simulink model "ThreeDOF_SMA_Spring_Hand"  (R2021b)
settings: Solver=FixedStepAuto  StartTime=0.0  StopTime=1.5  FixedStep=.001  RelTol=1e-3
libraries: RCTblocks x1
settings Model: Creator=Spino.shop  LastModifiedBy=Spino.shop
settings SFSimCC: SimTargetLang=C++

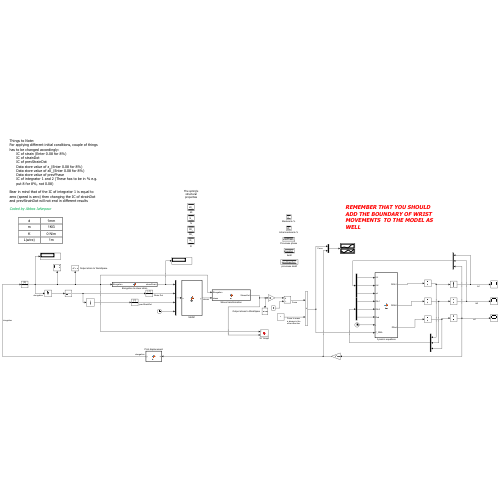
[thumbnail: Simulink's stored preview of the top-level diagram]
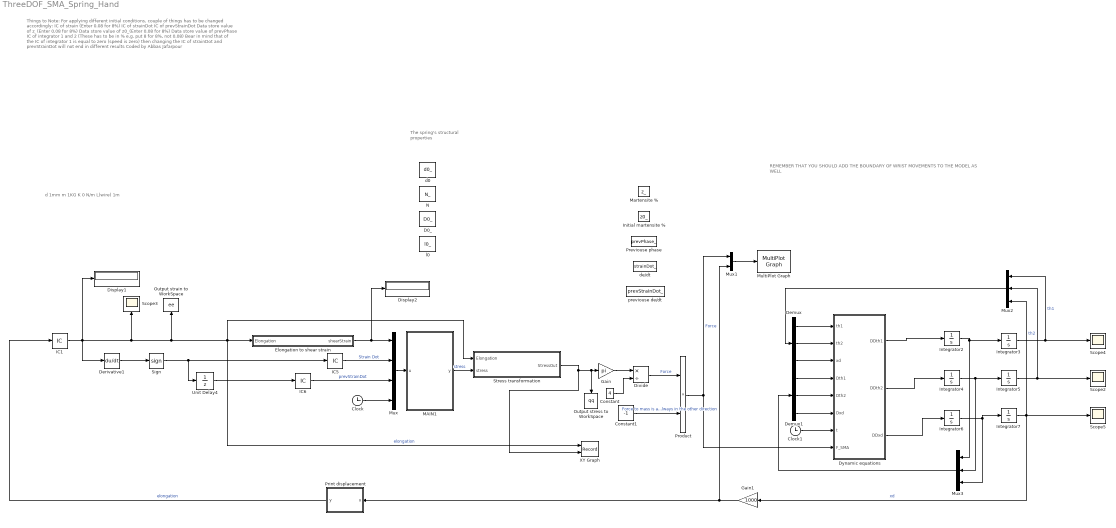
== system ThreeDOF_SMA_Spring_Hand ==
  note: Things to Note:
      | For applying different initial conditions, couple of things has to be changed accordingly:
      | IC of strain (Enter 0.08 for 8%)
      | IC of strainDot
      | IC of prevStrainDot
      | Data store value of z_(Enter 0.08 for 8%)
      | Data store value of z0_(Enter 0.08 for 8%)
      | Data store value of prevPhase
      | IC of integrator 1 and 2 (These has to be in % e.g. put 8 for 8%, not 0.08)
      |
      | Bear in mind that of the IC of integrator 1 is equal to zero (speed is zero) then changing the IC of strainDot and prevStrainDot will not end in different results
      |
      | Coded by Abbas Jafarpour
  note: d
      | 1mm
      |
      | m
      | 1KG
      |
      | K
      | 0 N/m
      |
      | L(wire)
      | 1m
  note: The spring's structural properties
  note: REMEMBER THAT YOU SHOULD ADD THE BOUNDARY OF WRIST MOVEMENTS TO THE MODEL AS WELL
  Clock : Clock
  Clock1 : Clock
  Constant : Constant  Value=4
  Constant1 : Constant  Value=-1
  D0_ : DataStoreMemory  DataStoreName=D0_  ReadBeforeWriteMsg=warning  WriteAfterWriteMsg=warning  WriteAfterReadMsg=warning  InitialValue=7.3  VectorParams1D=off  ShowAdditionalParam=off  OutDataTypeStr=double
  Demux : Demux  Outputs=3
  Demux1 : Demux  Outputs=3
  Derivative1 : Derivative
  Display1 : Display
  Display2 : Display
  Divide : Product  Inputs=*/
  Dynamic equations : MATLAB Function  TreatAsAtomicUnit=on
  Elongation to shear strain : MATLAB Function  TreatAsAtomicUnit=on
  Gain : Gain  Gain=pi
  Gain1 : Gain  Gain=1000
  IC1 : InitialCondition  Value=0
  IC5 : InitialCondition  Value=-1
  IC6 : InitialCondition  Value=-1
  Initial martensite % : DataStoreMemory  DataStoreName=z0_  ReadBeforeWriteMsg=warning  WriteAfterWriteMsg=warning  WriteAfterReadMsg=warning  InitialValue=1  ShowAdditionalParam=off  OutDataTypeStr=double
  Integrator{2..7} (6 alike) : Integrator
  MAIN1 : MATLAB Function  TreatAsAtomicUnit=on
  Martensite % : DataStoreMemory  DataStoreName=z_  ReadBeforeWriteMsg=warning  WriteAfterWriteMsg=warning  WriteAfterReadMsg=warning  InitialValue=0.015  ShowAdditionalParam=off  OutDataTypeStr=double
  MultiPlot Graph : RCTblocks/MultiPlot Graph  Tag=MultiPlot  tmin=0  tmax=1.5  ymin=-40  ymax=40  Tsamp=-1  vnamesave=multisimout
      settings: SourceProductBaseCode=RC
  Mux : Mux
  Mux1 : Mux  Inputs=2
  Mux2 : Mux  Inputs=3
  Mux3 : Mux  Inputs=3
  N : DataStoreMemory  DataStoreName=N_  ReadBeforeWriteMsg=warning  WriteAfterWriteMsg=warning  WriteAfterReadMsg=warning  InitialValue=5  ShowAdditionalParam=off  OutDataTypeStr=double
  Output strain to WorkSpace : ToWorkspace  VariableName=ee  SampleTime=-1
      settings: Save2DSignal=2-D array (concatenate along first dimension)
  Output stress to WorkSpace : ToWorkspace  VariableName=qq  SampleTime=-1
      settings: Save2DSignal=2-D array (concatenate along first dimension)
  Previouse phase : DataStoreMemory  DataStoreName=prevPhase_  ReadBeforeWriteMsg=warning  WriteAfterWriteMsg=warning  WriteAfterReadMsg=warning  InitialValue=5  ShowAdditionalParam=off  OutDataTypeStr=double
  Print displacement : MATLAB Function  TreatAsAtomicUnit=on
  Product : Product
  Scope{2..5} (4 alike) : Scope
  Sign : Signum
  Stress transformation : MATLAB Function  TreatAsAtomicUnit=on
  Unit Delay4 : UnitDelay  SampleTime=-1  HasFrameUpgradeWarning=on
  XY Graph : Record  FileSettingsInternal="{\"entries\":[{\"content\":{\"excelSettings\":{\"content\":{},\"type\":\"Streamout.ExcelSettings\"}},\"type\":\"Streamout.FileSettingStorage\",\"uuid\":\"8585d984-787d-4496-8735-ede648e09058\"}],\"packageUris\":[\"http://schema.mathworks.com/mf0/streamout_blocks/R2020a\"],\"version\":\"1.0\"}"  Layout=[1 1]  SignalsInternal="{\"entries\":[{\"content\":{\"signals\":[{\"content\":{\"blockPath\":[\"ThreeDOF_SMA_Spring_Hand/XY Graph\"],\"channel\":[],\"dimensions\":[1],\"domain\":\"ThreeDOF_SMA_Spring_Hand/XY Graph\",\"lineColor\":\"#a2142f\",\"plots\":[1],\"port\":1,\"sid\":[],\"signalID\":9,\"signalName\":\"elongation\"},\"type\":\"RecordBlkView.Signal\",\"uuid\":\"1176787e-02b1-4e58-a8f1-352873b659ce\"},{\"content\":{\"blockPath\":[\"ThreeDOF_SMA_Spring_Hand/XY Graph\"],\"channel\":[],\"dimensions\":[1],\"domain\":\"ThreeDOF_SMA_Spring_Hand/XY Graph\",\"lineColor\":\"#139fff\",\"plots\":[1],\"port\":2,\"sid\":[],\"signalID\":12,\"signalName\":\"Stress transformation\"},\"type\":\"RecordBlkView.Signal\",\"uuid\":\"6b0ce42b-1ab9-4c2f-8a20-9cf08699349f\"}]},\"type\":\"RecordBlkView.InputSignals\",\"uuid\":\"cd44c269-2911-4699-ac86-e4ccbff490f5\"}],\"packageUris\":[\"http://schema.mathworks.com/mf0/streamout_blocks/R2020a\"],\"version\":\"1.0\"}"  VisualizationBindings="{\"xyplotplugin\":{\"info\":[{\"series\":[{\"bindingParametersList\":[{\"parameter\":\"X-Axis\",\"signalID\":9,\"signalName\":\"elongation\"},{\"parameter\":\"Y-Axis\",\"signalID\":12,\"signalName\":\"Stress transformation\"}],\"seriesID\":6978}],\"subplotID\":1}]}}"  CompatibilityTag=XY
  d0 : DataStoreMemory  DataStoreName=d0_  ReadBeforeWriteMsg=warning  WriteAfterWriteMsg=warning  WriteAfterReadMsg=warning  InitialValue=1  ShowAdditionalParam=off  OutDataTypeStr=double
  de/dt : DataStoreMemory  DataStoreName=strainDot_  ReadBeforeWriteMsg=warning  WriteAfterWriteMsg=warning  WriteAfterReadMsg=warning  InitialValue=1  ShowAdditionalParam=off  OutDataTypeStr=double
  l0 : DataStoreMemory  DataStoreName=l0_  ReadBeforeWriteMsg=warning  WriteAfterWriteMsg=warning  WriteAfterReadMsg=warning  InitialValue=5  ShowAdditionalParam=off  OutDataTypeStr=double
  previouse de/dt : DataStoreMemory  DataStoreName=prevStrainDot_  ReadBeforeWriteMsg=warning  WriteAfterWriteMsg=warning  WriteAfterReadMsg=warning  InitialValue=1  ShowAdditionalParam=off  OutDataTypeStr=double
  wires:
  Unit Delay4/1 -> IC6/1
  Mux/1 -> MAIN1/1(u)
  Derivative1/1 -> Sign/1
  Clock/1 -> Mux/4
  Sign/1 -> Unit Delay4/1, IC5/1
  Gain/1 -> Divide/1
  Constant/1 -> Divide/2
  IC1/1 -> Scope3/1, Output strain to WorkSpace/1, Stress transformation/1(Elongation), XY Graph/1, Elongation to shear strain/1(Elongation), Derivative1/1, Display1/1  "elongation"
  IC5/1 -> Mux/2  "Strain Dot"
  IC6/1 -> Mux/3  "prevStrainDot"
  Divide/1 -> Product/1  "Force"
  Product/1 -> Dynamic equations/8(F_SMA), Mux1/1  "Force"
  Mux1/1 -> MultiPlot Graph/1
  Constant1/1 -> Product/2  "Force to mass is always in the other direction"
  Print displacement/1(y) -> IC1/1  "elongation"
  MAIN1/1(y) -> Stress transformation/2(stress)  "stress"
  Stress transformation/1(StressOut) -> XY Graph/2, Output stress to WorkSpace/1, Gain/1
  Elongation to shear strain/1(shearStrain) -> Display2/1, Mux/1
  Gain1/1 -> Mux1/2, Print displacement/1(u)
  Integrator2/1 -> Mux3/1, Integrator3/1
  Integrator6/1 -> Integrator7/1, Mux3/3
  Demux1/1 -> Dynamic equations/4(Dth1)
  Demux/3 -> Dynamic equations/3(xd)
  Mux2/1 -> Demux/1
  Demux1/2 -> Dynamic equations/5(Dth2)
  Integrator3/1 -> Scope4/1, Mux2/1  "th1"
  Dynamic equations/3(DDxd) -> Integrator6/1
  Demux/2 -> Dynamic equations/2(th2)
  Mux3/1 -> Demux1/1
  Demux/1 -> Dynamic equations/1(th1)
  Clock1/1 -> Dynamic equations/7(t)
  Integrator7/1 -> Gain1/1, Mux2/3, Scope5/1  "xd"
  Integrator5/1 -> Scope2/1, Mux2/2  "th2"
  Dynamic equations/1(DDth1) -> Integrator2/1
  Integrator4/1 -> Mux3/2, Integrator5/1
  Dynamic equations/2(DDth2) -> Integrator4/1
  Demux1/3 -> Dynamic equations/6(Dxd)

== matlab function ThreeDOF_SMA_Spring_Hand/Elongation to shear strain ==
  settings: updateMethod=DISCRETE
  data: shearStrain output; Elongation input; N_ data_store_memory; d0_ data_store_memory; D0_ data_store_memory; l0_ data_store_memory
% Because we have Nonlinear shera transformation in the entire
% crosssection, to avoide unncessary complexity we take shear as a linear
% function in the wire's crossection and approximate the integral. Refer to
% the paper for proof of the formula and the way we acquire these
% parameters.
function shearStrain = fcn(Elongation)
    
    % Processing the grlobal variables
    global D0_ d0_ l0_ N_;
    D0 = D0_;
    N = N_;
    d0 = d0_;
    l0 = l0_;

    R0 = D0/2;
    r0 = d0/2;

    alpha0 = atan(l0 / (2 * pi * N * R0) ); % Initial helix angle
    L = sqrt(l0 + (2 * pi * N * R0)^2); % The total length of the spring 
    
    r0  = d0 / 2;
    alpha = asin( Elongation / L + sin(alpha0) );
    R = R0 * cos(alpha) / cos(alpha0);
    
    shearStrain = Elongation * r0 / (2 * pi * N * R^2) * (3/4);
end

== matlab function ThreeDOF_SMA_Spring_Hand/Print displacement ==
  data: u input; y output
function y = fcn(u)
    y = u;
    fprintf("====>> displacement : %.5f\n",u);
end

== matlab function ThreeDOF_SMA_Spring_Hand/Stress transformation ==
  settings: updateMethod=DISCRETE
  data: Elongation input; stress input; StressOut output; N_ data_store_memory; l0_ data_store_memory; D0_ data_store_memory; d0_ data_store_memory
function StressOut = fcn(Elongation, stress)

    % Processing the grlobal variables
    global D0_ d0_ l0_ N_;
    D0 = D0_;
    N = N_;
    d0 = d0_;
    l0 = l0_;

    R0 = D0/2;
    r0 = d0/2;

    alpha0 = atan(l0 / (2 * pi * N * R0) ); % Initial helix angle
    L = sqrt(l0 + (2 * pi * N * R0)^2); % The total length of the spring 
    
    % Calculating the spring diameter change
    alpha = asin( Elongation / L + sin(alpha0) );
    R = R0 * cos(alpha) / cos(alpha0);

    StressOut = stress * 2 * pi * r0 ^ 3 / 3 / R;
end

== matlab function ThreeDOF_SMA_Spring_Hand/Dynamic equations ==
  data: th1 input; th2 input; xd input; Dth1 input; Dth2 input; Dxd input; DDth1 output; DDth2 output; DDxd output; t input; F_SMA input
function [DDth1, DDth2, DDxd] = fcn(th1, th2, xd, Dth1, Dth2, Dxd, t, F_SMA)

T1 = sin(t);
T2 = cos(t);


Y = zeros(6,1);
Y(1) = xd;
Y(2) = Dxd;
Y(3) = th1;
Y(4) = Dth1;
Y(5) = th2;
Y(6) = Dth2;

DDxd = -(3*F_SMA - T1 + cos(Y(3) - Y(5))^2*Y(2) - cos(Y(5))*cos(Y(3) - Y(5)) + sin(Y(3) - Y(5))*Y(6)^2 ...
    - sin(Y(3))*Y(1) + T2*cos(Y(3) - Y(5)) + cos(Y(3))*cos(Y(3) - Y(5))^2 - F_SMA*cos(Y(3) - Y(5))^2 ...
    - cos(Y(3) - Y(5))*Y(5) - cos(Y(3) - Y(5))*Y(6) - 3*Y(2) + Y(3) + Y(4) + ...
    cos(Y(3) - Y(5))*sin(Y(3) - Y(5))*Y(4)^2)/(cos(Y(3) - Y(5))^2 - 2);

DDth1 = (F_SMA - T1 + 2*cos(Y(3)) - cos(Y(5))*cos(Y(3) - Y(5)) + sin(Y(3) - Y(5))*Y(6)^2 - sin(Y(3))*Y(1) ...
    + T2*cos(Y(3) - Y(5)) - cos(Y(3) - Y(5))*Y(5) - cos(Y(3) - Y(5))*Y(6) - Y(2) + Y(3) + Y(4) + ...
    cos(Y(3) - Y(5))*sin(Y(3) - Y(5))*Y(4)^2)/(cos(Y(3) - Y(5))^2 - 2);

DDth2 = -(2*T2 - 2*cos(Y(5)) + 2*cos(Y(3))*cos(Y(3) - Y(5)) + 2*sin(Y(3) - Y(5))*Y(4)^2 + ...
    F_SMA*cos(Y(3) - Y(5)) - T1*cos(Y(3) - Y(5)) - cos(Y(3) - Y(5))*Y(2) + cos(Y(3) - Y(5))*Y(3) ...
    + cos(Y(3) - Y(5))*Y(4) - 2*Y(5) - 2*Y(6) + cos(Y(3) - Y(5))*sin(Y(3) - Y(5))*Y(6)^2 ...
    - sin(Y(3))*cos(Y(3) - Y(5))*Y(1))/(cos(Y(3) - Y(5))^2 - 2);

== matlab function ThreeDOF_SMA_Spring_Hand/MAIN1 ==
  settings: updateMethod=DISCRETE
  data: u input; y output; z_ data_store_memory; z0_ data_store_memory; prevPhase_ data_store_memory; d0_ data_store_memory; D0_ data_store_memory; l0_ data_store_memory; N_ data_store_memory
function y = fcn(u)

    % Processing the grlobal variables for Material structural
    % properties
    global D0_ d0_ l0_ N_;
    D0 = D0_; % Wire diameter (mm)
    N = N_  ; % Number of coils
    d0 = d0_; % Coil diameter (mm) 
    l0 = l0_; % Initial length of spring l0 (mm) 
        
    % Processing the grlobal variables for SMA phase and strain
    global z_ z0_ strainDot_ prevStrainDot_ prevPhase_;

    % Initiate material properties
    X = 6;
    if false
        kj = 1;
    elseif X == 6
        Mf = 9; Ms = 18.4; As = 34.5; Af = 49;
    
        CA_Loading = 13.8; CA_Unloading = 13.8;
        CM_Loading = 8   ; CM_Unloading = 8   ; 
        critStressFinish = 170; critStressStart = 100;
    
        Ga = 67e3; Gm = 26.3e3; eL = 0.067;
        T = 60;
    
        S_M_finish_Loading = critStressFinish + CM_Loading*(T-Ms); S_M_finish_Unloading = critStressFinish + CM_Unloading*(T-Ms);
        S_M_start_Loading = critStressStart + CM_Loading*(T-Ms); S_M_start_Unloading = critStressStart + CM_Unloading*(T-Ms);
        S_A_start_Loading = CA_Loading*(T-As); S_A_start_Unloading = CA_Unloading*(T-As);
        S_A_finish_Loading = CA_Loading*(T-Af); S_A_finish_Unloading = CA_Unloading*(T-Af);
    
        S_M_finish = [S_M_finish_Loading S_M_finish_Unloading];
        S_M_start = [S_M_start_Loading S_M_start_Unloading];
        S_A_start = [S_A_start_Loading S_A_start_Unloading];
        S_A_finish = [S_A_finish_Loading S_A_finish_Unloading];
    end


    y = 0;

    strain = u(1); eDot = u(2); prevStrainDot = u(3);
    
    % When eDot is zero, change eDot to previouse eDot
    if eDot == 0
        eDot = prevStrainDot;
    end

    % We get eDot from derivative of e with respect to time, on negative
    % strains this causes the code to think that we are unloading while
    % actually we are loading. we solve this by conditions below
    if(strain < 0 && eDot < 0)
        eDot = 1;
    elseif(strain < 0 && eDot > 0)
        eDot = -1;
    end

    % Do the same for previouse step's strainDot
    if(strain < 0 && prevStrainDot < 0)
        prevStrainDot = 1;
    elseif(strain < 0 && prevStrainDot > 0)
        prevStrainDot = -1;
    end

    fprintf("\n\nMAIN (%.4fs); z0:%.4f ||z:%.4f ||strain:%.5f || strainDot: %.1f || prevStrainDot: %.1f ||prevPhase:%.1f || \n",u(4), z0_,z_,strain,eDot,prevStrainDot,prevPhase_);
    % Note that: [z0,z,previousePahse,stress] --> [y(1),y(2),y(3),y(4)]

    [z0_,z_,prevPhase_,y] = MAIN(z0_,z_,prevPhase_,strain,eDot, prevStrainDot,T,eL,Gm,Ga,Ms,As, S_M_finish, S_M_start, S_A_finish, S_A_start);
    
    fprintf("One pass done.")

    y = double(y);

end

function [z0,z,phase,stress] = MAIN(z0,z,previousePahse,strain,strainDot, prevStrainDot,T,eL,Gm,Ga,Ms,As, S_M_finish, S_M_start, S_A_finish, S_A_start)
    coder.extrinsic("stressFinder");

    %This function with strain as an input and some other inputs, returns
    %stress and some other variables (These variables are used as inputs for the next iteration)
    %This function helps us avoide doing the calculations inside the loop
    %INPUTS:
    %z0: The martensite ratio at start of previouse phase
    %z: The martensite ratio of previouse iteration (It is different form z0)
    %prevPhase: The phase of previouse iteration
    %strain: Current strain
    %strainDot: Current strain rate

    %Only pseudoelastic
    zT = 0; zT0 = 0;

    %When we reverse in the middle of phase transformation, we need to
    %update z0, but due to us not having the stress, we cant know if we
    %have changed phase (phaseFinder function needs stress as an input)
    %to solve this error, we know if we have reversed if previose eDot
    %is not equal to current eDot. when they are not equal, we update
    %the value of z0
    reverse = false;
    if prevStrainDot ~= strainDot
        reverse = true;
    end

    if reverse
        zS0 = z;
        z0 = z;
    end
    
    % Passing different critical stress's to required functions for loading
    % and unlaoding. This helps us to adopt for the simulations that CM and
    % CA are different for loading and unloading
    if 0 <= strainDot
        i = 1;
    else
        i = 2;
    end

    stress = 0;
    stress = stressFinder(previousePahse, strain, strainDot, T, eL, Gm, Ga, z0, zT, S_M_finish(i), S_M_start(i), S_A_finish(i), S_A_start(i));

    phase = phaseFinder(previousePahse, stress, strainDot,z,z0, S_M_finish(i), S_M_start(i), S_A_finish(i), S_A_start(i));
    fprintf("Current phase: %.1f\n",phase);
    if previousePahse ~= phase
        phaseChange = true;
        fprintf("ER1\n");
    else
        phaseChange = false;
    end
    
    %When we finsh phase 2 and go to phase 3 z is not exactly equal to
    %1, this causes errors in stressFinder function, so by this line we
    %fix this
    if (previousePahse == 2 && phase == 3) || (previousePahse == 222 && phase == 3) 
        z = 1;
    elseif (previousePahse == 5 && phase == 6) 
        z = 0;
    end
    
    if phaseChange
        fprintf("ER2\n");
        zS0 = z;
        z0 = z;
    end

    %The get_z function cant process negative stresses, so we multiply the
    %stress by -1 and at the end we change it back
    if(strain < 0)
        fprintf("ER3\n");
        NEGATIVESTRAIN = true;
        stress = stress * -1;
    end

    z = get_z(stress,strainDot,T,Ms,As,z0,zT,z, S_M_finish(i), S_M_start(i), S_A_finish(i), S_A_start(i));
    
    %Change back
    if(strain < 0)
        fprintf("ER4\n");
        NEGATIVESTRAIN = true;
        stress = stress * -1;
    end

    z = double(z);
    z0 = double(z0);
    stress = double(stress);
end


function [phase] = phaseFinder(prevPhase, stress, strainDot,z,z0, S_M_finish, S_M_start, S_A_finish, S_A_start)
    %Note that due to nature of my project zT is always equal to zero and we can use z instead of zS
    stress = double(stress);

    %This function returns the SMA's phase number in pseudoelastic a
    %procedure with Brinsons's (1993 and 1996) constitutive modeling
    %Phase Numbering:
    %loading before phase change : 1  || loading with phase change : 2  || loading after phase change : 3 
    %unloading before phase change : 4  || unloading with phase change : 5  || unloading after phase change : 6 
    %Phases for handeling inner loops are:
    %Loading while in middle of Martensite->Austenite phase change: 8
    %Loading when below martensit transformation start stress while  z != 0: 9
    %Loading while coming back into austenite phase Chaneg area while  z !=0: 10
    %**Note that the phases that are caused from reversals in loading in the middle of  a phase are repeated numers (e.g. 77 or 11)
    %Unloading before Austenite has changed to martensite (reversing in middle of phase 1):11
    %Unloading while in middle of Austenite->Martensite phase change: 22
    %Reversing phase 7 and continuing loading:77
    %Reversing in middle of phase 5 and continuing loading:55
    %
    %
    %For defining the inner loops we also need to know where we came from,
    %so we need the previous step's direction (loading or unloading)
    %* Note that stressDot is the direction of loading, +1 for loading and
    %-1 for unloading

    %UPDATE: some times, we have negative strain. In order for this
    %function to handle that, we define This constant. if it is true, all
    %the calculations will be in positive numbers but at the end they will
    %be multiplied by -1
    NEGATIVESTRAIN = false;
    
    if(stress < 0)
        NEGATIVESTRAIN = true;
        stress = stress * -1;
    end

    phase = -1;
    if (S_M_start < stress && stress < S_M_finish) && 0 < strainDot && z0 == 0
        phase = 2;
    elseif not(S_M_start < stress && stress < S_M_finish) && (stress < S_M_start) && 0 < strainDot && z == 0
        phase = 1;
    elseif not(S_M_start < stress && stress < S_M_finish) && (S_M_finish < stress) && 0 < strainDot
        phase = 3;
    elseif not( S_A_finish < stress && stress < S_A_start  ) && strainDot < 0 && (S_A_start < stress)  && z == 1
        phase = 4;
    elseif ( S_A_finish < stress && stress < S_A_start  ) && strainDot < 0 && 0 < z
        phase = 5;
    elseif not( S_A_finish < stress && stress < S_A_start  ) && strainDot < 0  && (stress < S_A_finish) && prevPhase ~= 11
        %Some times we start unloading while in phase 1, so to
        %differenciate this with phase 6, we have to make a new phase and
        %"&& prevPhase ~= 1" condition as well. to avoid devision by zero
        %add
        phase = 6;
    elseif not(S_M_start < stress && stress < S_M_finish) && (stress < S_M_start) && strainDot < 0 && z == 0
        %Unloading before Austenite has changed to martensite (reversing in middle of phase 1)
        phase = 11;
    elseif (z0 < 1) && (stress < S_M_finish) && (S_A_start < stress) && strainDot < 0
        %Inner loop: Unloading while in middle of Austenite->Martensite phase change
        phase = 22;
    elseif ( S_A_finish < stress && stress < S_A_start  ) && 0 < strainDot && 0 < z
        phase = 55;
    elseif (0 < z0) && (z0 < 1) && (stress < S_M_finish) && (S_A_start < stress) && 0 < strainDot
        %Inner loop: Reversing phase 22 and continuing loading
        phase = 222;
    elseif ( S_A_finish < stress && stress < S_A_start  ) && strainDot < 0 && z < 1
        %Inner loop: Unloading Phase transform from a point where z < 1
        phase = 8;
    elseif (S_M_start < stress && stress < S_M_finish) && 0 < strainDot && 0 < z
        %Inner loop: Loading while coming back into austenite phase Chaneg area while  z !=0
        phase = 10;
    end

end

function [z] = get_z(stress,stressDot,T,Ms,As,zS0,zT0,currZ, S_M_finish, S_M_start, S_A_finish, S_A_start)
    %This function returns total martensite ratio
    z = -99;
    if 0 < stressDot
        %Loading
        [z,~,~] = Func_Brinson_Conversion_To_Detwinned_Martensite(T,stress,Ms,zS0,zT0, S_M_finish, S_M_start, S_A_finish, S_A_start);
    elseif stressDot == 0
        z = -9999999;
    elseif stressDot < 0
        %Unloading
        [z,~,~] = Func_Brinson_Conversion_To_Austenite(T,stress,As,zS0,zT0,currZ, S_M_finish, S_M_start, S_A_finish, S_A_start);
    end
end


function [z,zS,zT] = Func_Brinson_Conversion_To_Austenite(T,stress,As,zS0,zT0,currZ, S_M_finish, S_M_start, S_A_finish, S_A_start)
    %This function returns the amount of stress induced and tempreature induced
    %Martensite in the process of SMA's conversion to austenite.
    %The brinson's 1993 constitutive relation has been used
    %z0 : martensite ration in the beginning of loading cycle
    %zT0 : temprature induced martensite ration in the beginning of loading cycle
    %zS0 : Stress induced martensite ration in the beginning of loading cycle
    %currZ: Current martensite ratio of the sample; thiw helps us to avoid
    %division by zero in phase 11
    %Note that Af < T
    %Note that this relation stands true only if: CA*(T-As) < stress < CA*(T-Af)
    %Also note that phase transformation from Martensite to Austenite
    %happens only when specimen is in the "Unloading" phase and stress is
    %decreasing (zDot < 0)

    % Update: in this update we removed the criticalStressStart and
    % criticalStressFinish from the required arguments. the user has to
    % only provide S_A_start and S_A_finish (Critical stress that
    % conversion to austenite starts and ends respectivelt). the user has
    % to calculate these parameters and pass them to method. In some papers
    % there is no criticalStress provided (unlike the brinson's model. we use
    % this method to make the function more friendly for implementing other
    % papaers)
    if (As < T) && (S_A_finish < stress && stress < S_A_start )
        if 0 < currZ
            z0 = zT0 + zS0;
            z = z0/2*(cos( pi/(S_A_start-S_A_finish)*(stress-S_A_start) )+1);
            zS = zS0 - zS0/z0*(z0-z);
            zT = zT0 - zT0/z0*(z0-z);
        else
            zS = zS0;
            zT = zT0;
            z = zS + zT;
        end
        
    else
        zS = zS0;
        zT = zT0;
        z = zS + zT;
    end
end


function [z,zS,zT] = Func_Brinson_Conversion_To_Detwinned_Martensite(T,stress,Ms,zS0,zT0, S_M_finish, S_M_start, S_A_finish, S_A_start)
    %This function returns the amount of stress induced and tempreature induced
    %Martensite in the process of SMA's conversion to detwinned martensite.
    %The brinson's 1993 constitutive relation has been used
    %z0 : martensite ration in the beginning of loading cycle
    %zT0 : temprature induced martensite ration in the beginning of loading cycle
    %zS0 : Stress induced martensite ration in the beginning of loading cycle
    %Note that Ms < T
    %Note that this relation stands true only if: 
    %criticalStressStart + CM*(T-Ms) < stress < criticalStressFinisg + CM*(T-Ms)
    %Also note that phase transformation from austenite to detwinned martensite
    %happens only when specimen is in the "Loading" phase and stress is
    %increasing (0 < zDot)

    % Update: in this update we removed the criticalStressStart and
    % criticalStressFinish from the required arguments. the user has to
    % only provide S_M_start and S_M_finish (Critical stress that
    % conversion to austenite starts and ends respectivelt). the user has
    % to calculate these parameters and pass them to method. In some papers
    % there is no criticalStress provided (unlike the brinson's model. we use
    % this method to make the function more friendly for implementing other
    % papaers)
    if (Ms < T) && (S_M_start < stress && stress < S_M_finish)
        zS = (1-zS0)/2*cos(pi/(S_M_start - S_M_finish) * (stress - S_M_finish)) + (1 + zS0)/2;
        zT = zT0 - zT0 / (1-zT0) * (zS - zS0);
        z = zS + zT;
    else
        zS = zS0;
        zT = zT0;
        z = zS + zT;
    end
end
